simulink model "NN Controlled IM Drive"  (R2020b)
settings: Solver=ode4  StartTime=0.0  StopTime=5  RelTol=1e-3
InitFcn:
  | %clear;
  | %clc;
  | 
  | %Motor Parameters
  | r1 = 1.405;
  | l1  = 0.005839;
  | r2 = 1.395;
  | l2 = 0.005839;
  | Lm = 0.1722;
  | J = 0.0131;
  | 
  | %Motor Rated Values
  | Vrat = 400;
  | frat = 50;
  | 
  | x1 = 2*pi*frat*l1;
  | x2 = 2*pi*frat*l2;
  | Xm = 2*pi*frat*Lm;
  | Prat = 4*1000;
  | Nrat = 1430;
  | P = 4;
  | Ns = 120*frat/P;
  | nrat = Nrat*2*pi/60;
  | ns = Ns*2*pi/60;
  | srat = (Ns-Nrat)/Ns;
  | 
  | E1 = Vrat/sqrt(3); %phase voltage
  | IL = E1/( (r1 + (1i*x1) ) + ( ( (1i*x2) +(r2/srat) )*1i*Xm / ( (1i*Xm) + (1i*x2) + (r2/srat) ) ) );
  | E2 = E1 - (IL*(r1 + (1i*x1) ) );
  | Trat = (3/(ns))*srat*abs(E2)*abs(E2)*r2/((r2*r2) + (srat*srat*x2*x2));
  | %Trat = Prat/nrat;
  | 
  | %System Variables
  | Tsys = (1e-6);
  | Ts = (100e-6);
  | freq = 50;
  | ws = freq*2*pi;
  | 
  | m=1*freq/50;
  | %m = 1 * (freq/50);
  | Vbus = (400*sqrt(2)*2/sqrt(3)) / (1.15);
  | 
  | Vref = (Vbus*sqrt(3)/2) * m;
  | delay = Ts/Tsys;
  | 
  | % Motor Starting Parameters
  | inc_time = 0.1;
  | 
  | %Motor Loading time
  | load_time = 0;
  | 
  | %No. of Hybrid Zones
  | numzones = 3;
  | 
  | %Load ML model Weights
  | 
  | W1R_s1 = readmatrix('Regression Weights\W1_subnet1_tmp_odd_90.xlsx');
  | b1R_s1 = readmatrix('Regression Weights\b1_subnet1_tmp_odd_90.xlsx');
  | W1R_s2 = readmatrix('Regression Weights\W1_subnet2_tmp_odd_90.xlsx');
  | b1R_s2 = readmatrix('Regression Weights\b1_subnet2_tmp_odd_90.xlsx');
  | 
  | W2R = readmatrix('Regression Weights\W2_subnet_tmp_odd_90.xlsx');
  | b2R = readmatrix('Regression Weights\b2_subnet_tmp_odd_90.xlsx');
  | 
  | 
  | W1C_s1 = readmatrix('Classification Weights\W1_subnet1_tmp.xlsx');
  | b1C_s1 = readmatrix('Classification Weights\b1_subnet1_tmp.xlsx');
  | W1C_s2 = readmatrix('Classification Weights\W1_subnet2_tmp.xlsx');
  | b1C_s2 = readmatrix('Classification Weights\b1_subnet2_tmp.xlsx');
  | 
  | W2C = readmatrix('Classification Weights\W2_subnet_tmp.xlsx');
  | b2C = readmatrix('Classification Weights\b2_subnet_tmp.xlsx');
  | 
  | %For Vector Control
  | Ls = l1+Lm;
  | Lr = l2+Lm;
  | Tr = Ls/r2;
  | w_s = Ns*2*pi/60;
  | sigma = 1-(Lm*Lm/(Ls*Lr));
  | sigma_r = (Lr/Lm)-1;
  | G = 1;
  | 
  | %isd_star = 3.9346;
  | %isq_star = 7.5149;
  | w_star = nrat;
  | %phi_star = 0.7005;
  | 
  | T = (Prat/nrat);
  | isd_star = Vrat*sqrt(2/3)/sqrt((r1.^2)+((2*pi*frat*Ls).^2));
  | phi_star = Lm*isd_star;
  | cnst = (3/2)*(P/2)*(Lm*Lm/Lr)*isd_star;
  | isq_star = T/cnst;
  | 
  | %Load Controller NN Weights \tmp14_++
  | W1_c = readmatrix('Controller NN Weights\tmp14_++\W1.xlsx');
  | b1_c = readmatrix('Controller NN Weights\tmp14_++\b1.xlsx');
  | W2_c = readmatrix('Controller NN Weights\tmp14_++\W2.xlsx');
  | b2_c = readmatrix('Controller NN Weights\tmp14_++\b2.xlsx');
  | 
  | %Speed Control Loop
  | tau = 0.318e-3;
  | K_cont = (2/3)*(P/2)*(1/(1+sigma_r))*phi_star;
  | Ksp = J/(2*K_cont*tau);
  | Ksi = 1/(4*tau);
  | 
  | %ZOH Time
  | Tzoh = 1e-4;
undefined symbols (not defined in the file): DiscIntNeverNeededParam
libraries: powerlib x22, simulink x20, pid_lib x4, powerlib_meascontrol x3, simulink_extras x2
(part 1 of 3)
settings Model: Creator=hp  LastModifiedBy=hp
settings DataIOCC: ReturnWorkspaceOutputs=off

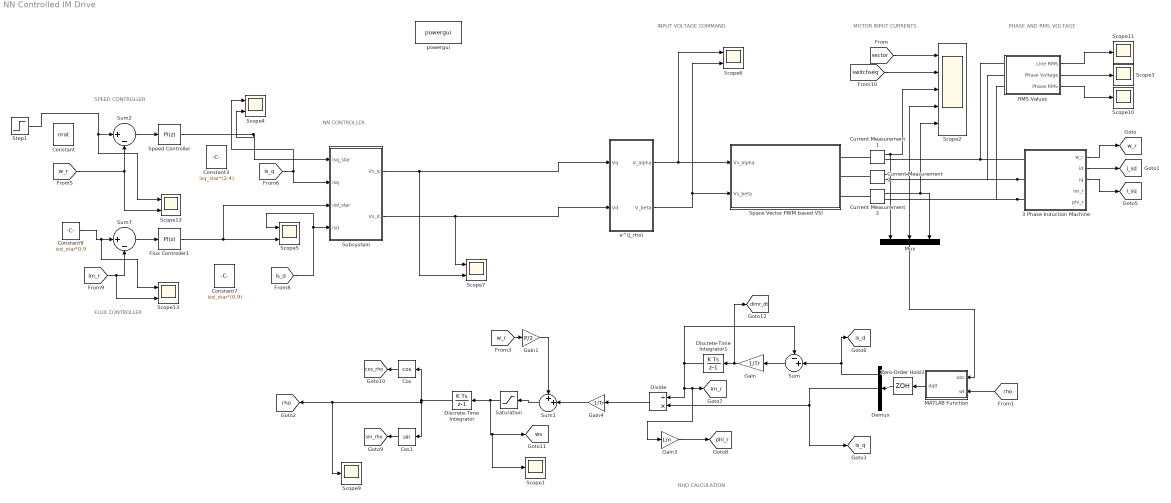
== system NN Controlled IM Drive ==
  note: PHASE AND RMS VOLTAGE
  note: MOTOR INPUT CURRENTS
  note: RHO CALCULATION
  note: INPUT VOLTAGE COMMAND
  note: NN CONTROLLER
  note: FLUX CONTROLLER
  note: SPEED CONTROLLER
  3 Phase Induction Machine : Subsystem
  Constant : Constant  Value=nrat
  Constant3 : Constant  Value=isq_star*(2.4)
  Constant7 : Constant  Value=isd_star*(0.9)
  Constant9 : Constant  Value=isd_star*0.9
  Cos : Trigonometry  Operator=cos
  Cos1 : Trigonometry
  Current Measurement1 : powerlib/Measurements/Current Measurement  PhasorSimulation=off  OutputType=Complex  PSBequivalent=0
  Current Measurement2 : powerlib/Measurements/Current Measurement  PhasorSimulation=off  OutputType=Complex  PSBequivalent=0
  Current Measurement3 : powerlib/Measurements/Current Measurement  PhasorSimulation=off  OutputType=Complex  PSBequivalent=0
  Demux : Demux  Outputs=3
  Discrete-Time Integrator : DiscreteIntegrator  SampleTime=-1  ICPrevOutput=DiscIntNeverNeededParam  ICPrevScaledInput=DiscIntNeverNeededParam
  Discrete-Time Integrator1 : DiscreteIntegrator  InitialCondition=1e-2  SampleTime=-1  ICPrevOutput=DiscIntNeverNeededParam  ICPrevScaledInput=DiscIntNeverNeededParam
  Divide : Product  Inputs=/*
  Flux Controller1 : pid_lib/PID Controller  Controller=PI  Form=Ideal  TimeDomain=Discrete-time  UseExternalTs=off  SampleTime=-1  IntegratorMethod=Forward Euler  FilterMethod=Forward Euler  ControllerParametersSource=internal  P=16*0.5*1.5/0.5  I=0.5*10/10  D=0  UseFilter=on  N=100  TunerSelectOption=Transfer Function Based (PID Tuner App)  InitialConditionSource=internal  InitialConditionForIntegrator=0  InitialConditionForFilter=0  DifferentiatorICPrevScaledInput=0  ExternalReset=none  TrackingMode=off  Kt=1  LimitOutput=on  SatLimitsSource=internal  UpperSaturationLimit=7  LowerSaturationLimit=-7  LinearizeAsGain=on  AntiWindupMode=none  Kb=1  POutMin=[]  POutMax=[]  IOutMin=[]  IOutMax=[]  DOutMin=[]  DOutMax=[]  NOutMin=[]  NOutMax=[]  SumOutMin=[]  SumOutMax=[]  SaturationOutMin=[]  SaturationOutMax=[]  PParamMin=[]  PParamMax=[]  IParamMin=[]  IParamMax=[]  DParamMin=[]  DParamMax=[]  NParamMin=[]  NParamMax=[]  KbParamMin=[]  KbParamMax=[]  KtParamMin=[]  KtParamMax=[]  KbOutMin=[]  KbOutMax=[]  KtOutMin=[]  KtOutMax=[]  IntegratorOutMin=[]  IntegratorOutMax=[]  FilterOutMin=[]  FilterOutMax=[]  SumI1OutMin=[]  SumI1OutMax=[]  SumI2OutMin=[]  SumI2OutMax=[]  SumI3OutMin=[]  SumI3OutMax=[]  SumI4OutMin=[]  SumI4OutMax=[]  SumDOutMin=[]  SumDOutMax=[]  DifferentiatorOutMin=[]  DifferentiatorOutMax=[]  FilterDiffOutCoefMin=[]  FilterDiffOutCoefMax=[]  ReciprocalOutMin=[]  ReciprocalOutMax=[]  SumDenOutMin=[]  SumDenOutMax=[]  SumNumOutMin=[]  SumNumOutMax=[]  DivideOutMin=[]  DivideOutMax=[]  UdiffTsProdOutMin=[]  UdiffTsProdOutMax=[]  NTsProdOutMin=[]  NTsProdOutMax=[]  UintegralTsProdOutMin=[]  UintegralTsProdOutMax=[]  UngainTsProdOutMin=[]  UngainTsProdOutMax=[]  IntegratorContinuousStateAttributes=''  IntegratorStateMustResolveToSignalObject=off  IntegratorRTWStateStorageClass=Auto  FilterContinuousStateAttributes=''  FilterStateMustResolveToSignalObject=off  FilterRTWStateStorageClass=Auto  ParallelPVariant=Passthrough  IdealPVariant=InternalParameters  IVariant=InternalParameters  DVariant=Disabled  IntegratorVariant=Discrete  SatVariant=Enabled  AWVariant=Passthrough  PCopyVariant=Disabled  TRVariant=Disabled  FdbkBlocksVariant=Forward  IdealPFdbkVariant=Disabled  SatFdbkVariant=Disabled  DerivativeFilterVariant=Disabled  NVariant=Disabled  NCopyVariant=Disabled_SignalSpec  FilterICVariant=Disabled  IntegratorICVariant=InternalICs  ExternalResetVariant=Disabled  TRSumVariant=Passthrough  SumFdbkVariant=Disabled  SumVariant=Sum_PI  TsampFilterVariant=InternalTs  TsampNgainVariant=Passthrough  TsampIntegralVariant=Passthrough  ExternalSaturationOutDataTypeStr=Inherit: Same as second input
  Gain : Gain  Gain=1/Tr
  Gain1 : Gain  Gain=P/2
  Gain3 : Gain  Gain=Lm
  Gain4 : Gain  Gain=1/Tr
  MATLAB Function : MATLAB Function  TreatAsAtomicUnit=on
  Mux : Mux  Inputs=3
  RMS Values : Subsystem
  Saturation : Saturate  UpperLimit=2*ws  LowerLimit=-2*ws
  Scope{1,3,9..11} (5 alike) : Scope
  Scope{4..7,12..13} (6 alike) : Scope  NumInputPorts=2
  Scope2 : Scope  NumInputPorts=5
  "Space Vector PWM based VSI " : Subsystem
  Speed Controller : pid_lib/PID Controller  Controller=PI  Form=Ideal  TimeDomain=Discrete-time  UseExternalTs=off  SampleTime=-1  IntegratorMethod=Forward Euler  FilterMethod=Forward Euler  ControllerParametersSource=internal  P=0.11*2/2  I=10*5/5  D=0  UseFilter=on  N=100  TunerSelectOption=Transfer Function Based (PID Tuner App)  InitialConditionSource=internal  InitialConditionForIntegrator=0  InitialConditionForFilter=0  DifferentiatorICPrevScaledInput=0  ExternalReset=none  TrackingMode=off  Kt=1  LimitOutput=on  SatLimitsSource=internal  UpperSaturationLimit=30  LowerSaturationLimit=-14  LinearizeAsGain=on  AntiWindupMode=none  Kb=1  POutMin=[]  POutMax=[]  IOutMin=[]  IOutMax=[]  DOutMin=[]  DOutMax=[]  NOutMin=[]  NOutMax=[]  SumOutMin=[]  SumOutMax=[]  SaturationOutMin=[]  SaturationOutMax=[]  PParamMin=[]  PParamMax=[]  IParamMin=[]  IParamMax=[]  DParamMin=[]  DParamMax=[]  NParamMin=[]  NParamMax=[]  KbParamMin=[]  KbParamMax=[]  KtParamMin=[]  KtParamMax=[]  KbOutMin=[]  KbOutMax=[]  KtOutMin=[]  KtOutMax=[]  IntegratorOutMin=[]  IntegratorOutMax=[]  FilterOutMin=[]  FilterOutMax=[]  SumI1OutMin=[]  SumI1OutMax=[]  SumI2OutMin=[]  SumI2OutMax=[]  SumI3OutMin=[]  SumI3OutMax=[]  SumI4OutMin=[]  SumI4OutMax=[]  SumDOutMin=[]  SumDOutMax=[]  DifferentiatorOutMin=[]  DifferentiatorOutMax=[]  FilterDiffOutCoefMin=[]  FilterDiffOutCoefMax=[]  ReciprocalOutMin=[]  ReciprocalOutMax=[]  SumDenOutMin=[]  SumDenOutMax=[]  SumNumOutMin=[]  SumNumOutMax=[]  DivideOutMin=[]  DivideOutMax=[]  UdiffTsProdOutMin=[]  UdiffTsProdOutMax=[]  NTsProdOutMin=[]  NTsProdOutMax=[]  UintegralTsProdOutMin=[]  UintegralTsProdOutMax=[]  UngainTsProdOutMin=[]  UngainTsProdOutMax=[]  IntegratorContinuousStateAttributes=''  IntegratorStateMustResolveToSignalObject=off  IntegratorRTWStateStorageClass=Auto  FilterContinuousStateAttributes=''  FilterStateMustResolveToSignalObject=off  FilterRTWStateStorageClass=Auto  ParallelPVariant=Passthrough  IdealPVariant=InternalParameters  IVariant=InternalParameters  DVariant=Disabled  IntegratorVariant=Discrete  SatVariant=Enabled  AWVariant=Passthrough  PCopyVariant=Disabled  TRVariant=Disabled  FdbkBlocksVariant=Forward  IdealPFdbkVariant=Disabled  SatFdbkVariant=Disabled  DerivativeFilterVariant=Disabled  NVariant=Disabled  NCopyVariant=Disabled_SignalSpec  FilterICVariant=Disabled  IntegratorICVariant=InternalICs  ExternalResetVariant=Disabled  TRSumVariant=Passthrough  SumFdbkVariant=Disabled  SumVariant=Sum_PI  TsampFilterVariant=InternalTs  TsampNgainVariant=Passthrough  TsampIntegralVariant=Passthrough  ExternalSaturationOutDataTypeStr=Inherit: Same as second input
  Step1 : Step  Time=0.5  After=nrat  SampleTime=0
  Subsystem : Subsystem
  Sum : Sum  Inputs=-+|
  Sum1 : Sum  Inputs=++|
  Sum2 : Sum  Inputs=|+-
  Sum7 : Sum  Inputs=|+-
  Zero-Order Hold3 : ZeroOrderHold  SampleTime=Tzoh
  e^(j_rho) : Subsystem
  powergui : powerlib/powergui  Priority=1  SimulationMode=Discrete  SampleTime=1e-6  frequency=60  Iterations=50  frequencyindice=50  Pbase=100e6  ErrMax=1e-4  UnitsV=kV  UnitsW=MW  buscounter=0  FunctionMessages=off  echomessages=off  EnableUseOfTLC=off  CurrentSourceSwitches=off  DisableSnubberDevices=off  DisableRonSwitches=off  DisableVfSwitches=off  DisplayEquations=off  AutomaticDiscreteSolvers=off  SolverType=Tustin/Backward Euler (TBE)  Interpol=off  ExternalGateDelay=off  methode=off  Ts=100  x0status=blocks  SPID=on  SwTol=0  HookPort=off  NonlinearTolerance=1e-4  nMaxIteration=100  ContinueOnMaxIteration=off  RestoreLinks=warning  ResistiveCurrentMeasurement=off  Frange=[0:2:500]  Ylog=off  Xlog=on  ShowGrid=off  save=off  variable=ZData  structure=ScopeData4  ZoomFFT=off  StartTime=1.4  cycles=1  DisplayStyle=1  fundamental=50  FreqAxis=off  MaxFrequency=1000  frequencyindicesteady=1  RmsSteady=1  display=off
  tag scope: cos_rho=global, dimr_dt=global, i_sd=global, i_sq=global, im_r=global, is_d=global, is_q=global, phi_r=global, rho=global, sin_rho=global, w_r=global, ws=global
  wires:
  Current Measurement2/1 -> Mux/2, Scope2/4
  3 Phase Induction Machine/1(w_r) -> [w_r]
  e^(j_rho)/2(V_beta) -> Scope6/2, "Space Vector PWM based VSI "/2(Vs_beta)
  Discrete-Time Integrator1/1 -> Sum/1, Gain3/1, [im_r], Divide/1
  [rho] -> MATLAB Function/2(wt)
  Mux/1 -> MATLAB Function/1(abc)
  [w_r] -> Gain1/1
  Demux/1 -> [is_d], Sum/2
  [switchseq] -> Scope2/2
  Gain/1 -> [dimr_dt], Discrete-Time Integrator1/1
  e^(j_rho)/1(V_alpha) -> Scope6/1, "Space Vector PWM based VSI "/1(Vs_alpha)
  Sum/1 -> Gain/1
  Demux/2 -> [is_q], Divide/2
  Current Measurement1/1 -> Scope2/3, Mux/1
  Cos1/1 -> [sin_rho]
  Current Measurement3/1 -> Mux/3, Scope2/5
  Gain1/1 -> Sum1/1
  [im_r] -> Scope13/2, Sum7/2
  [w_r] -> Sum2/2, Scope12/2
  RMS Values/1(Line RMS) -> Scope11/1
  Sum2/1 -> Speed Controller/1
  3 Phase Induction Machine/2(id) -> [i_sd]
  Sum7/1 -> Flux Controller1/1
  Discrete-Time Integrator/1 -> Scope9/1, [rho], Cos1/1, Cos/1
  3 Phase Induction Machine/3(iq) -> [i_sq]
  RMS Values/3(Phase RMS) -> Scope10/1
  RMS Values/2(Phase Voltage) -> Scope3/1
  Cos/1 -> [cos_rho]
  [sector] -> Scope2/1
  Sum1/1 -> Saturation/1
  Saturation/1 -> Scope1/1, [ws], Discrete-Time Integrator/1
  Constant9/1 -> Scope13/1, Sum7/1
  Step1/1 -> Scope12/1, Sum2/1
  Gain3/1 -> [phi_r]
  Gain4/1 -> Sum1/2
  Divide/1 -> Gain4/1
  MATLAB Function/1(dq0) -> Zero-Order Hold3/1
  [is_q] -> Scope4/1, Subsystem/2(isq)
  [is_d] -> Scope5/1, Subsystem/4(isd)
  Subsystem/2(Vs_d) -> e^(j_rho)/2(Vd), Scope7/1
  Subsystem/1(Vs_q) -> e^(j_rho)/1(Vq), Scope7/2
  Speed Controller/1 -> Scope4/2, Subsystem/1(isq_star)
  Flux Controller1/1 -> Subsystem/3(isd_star), Scope5/2
  Zero-Order Hold3/1 -> Demux/1
  connections:
  3 Phase Induction Machine/LConn2 -- RMS Values/LConn2 -- Current Measurement2/RConn1
  RMS Values/LConn1 -- Current Measurement1/RConn1 -- 3 Phase Induction Machine/LConn1
  3 Phase Induction Machine/LConn3 -- RMS Values/LConn3 -- Current Measurement3/RConn1
  Current Measurement1/LConn1 -- "Space Vector PWM based VSI "/RConn1
  Current Measurement3/LConn1 -- "Space Vector PWM based VSI "/RConn3
  Current Measurement2/LConn1 -- "Space Vector PWM based VSI "/RConn2

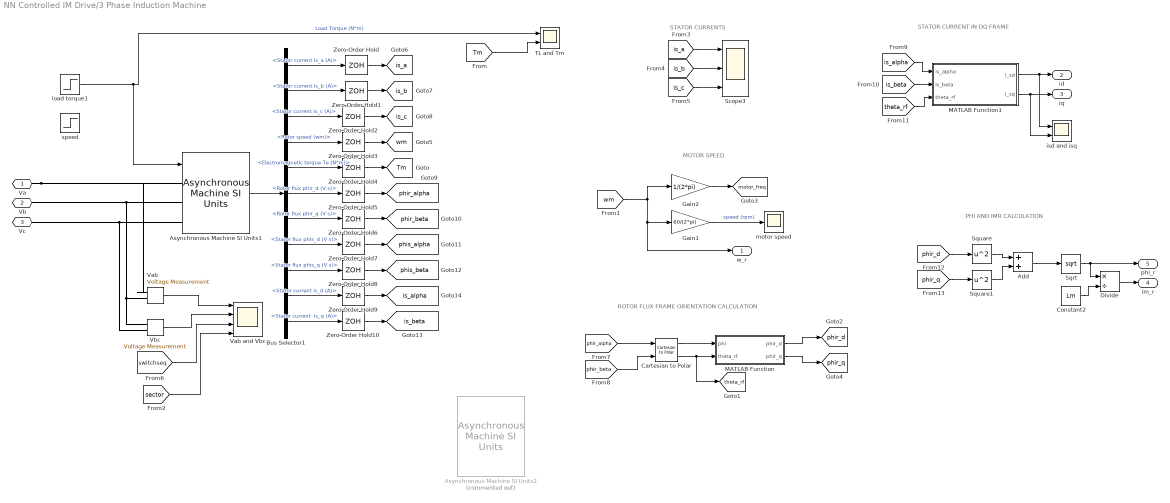
== system NN Controlled IM Drive/3 Phase Induction Machine ==
  note: MOTOR SPEED
  note: STATOR CURRENTS
  note: ROTOR FLUX FRAME ORIENTATION CALCULATION
  note: STATOR CURRENT IN DQ FRAME
  note: PHI AND IMR CALCULATION
  Add : Sum
  Asynchronous Machine SI Units1 : powerlib/Machines/Asynchronous Machine SI Units  RotorType=Squirrel-cage  PresetModel=No  MechanicalLoad=Torque Tm  ShowDetailedParameters=on  ReferenceFrame=Stationary  Units=SI  MeasurementBus=off  NominalParameters=[4000 400 50]  Stator=[1.405 0.005839]  Rotor=[1.395 0.005839]  Cage1=[0.4155 0.002066]  Cage2=[0.4168 0.0003495]  Lm=0.1722  Mechanical=[0.02 0.002985 2]  PolePairs=2  InitialConditions="[ 1,0   0,0,0   0,0,0 ]"  SimulateSaturation=off  Saturation=[14.03593122, 27.81365428, 53.79336849, 72.68890987, 97.98006896, 148.6815601, 215.7428561, 302.9841135, 428.7778367 ; 230, 322, 414, 460, 506, 552, 598, 644, 690]  LoadFlowParameters=1492000  TsPowergui=0  TsBlock=-1  IterativeModel=Trapezoidal non iterative  IterativeDiscreteModel=Trapezoidal non iterative  Pmec=0
  Asynchronous Machine SI Units2 : powerlib/Machines/Asynchronous Machine SI Units  Commented=on  RotorType=Squirrel-cage  PresetModel="15:  5.4 HP (4KW)   400 V  50Hz 1430 RPM"  MechanicalLoad=Torque Tm  ShowDetailedParameters=on  ReferenceFrame=Stationary  Units=SI  MeasurementBus=off  NominalParameters=[4000 400 50]  Stator=[1.405 0.005839]  Rotor=[1.395 0.005839]  Cage1=[0.4155 0.002066]  Cage2=[0.4168 0.0003495]  Lm=0.1722  Mechanical=[0.0131 0.002985 2]  PolePairs=2  InitialConditions="[ 1,0   0,0,0   0,0,0 ]"  SimulateSaturation=off  Saturation=[14.03593122, 27.81365428, 53.79336849, 72.68890987, 97.98006896, 148.6815601, 215.7428561, 302.9841135, 428.7778367 ; 230, 322, 414, 460, 506, 552, 598, 644, 690]  LoadFlowParameters=1492000  TsPowergui=0  TsBlock=-1  IterativeModel=Trapezoidal non iterative  IterativeDiscreteModel=Trapezoidal non iterative  Pmec=0
  Bus Selector1 : BusSelector  OutputSignals="Stator measurements.Stator current is_a (A),Stator measurements.Stator current is_b (A),Stator measurements.Stator current is_c (A),Mechanical.Rotor speed (wm),Mechanical.Electromagnetic torque Te (N*m),Rotor measurements.Rotor flux phir_d (V s),Rotor measurements.Rotor flux phir_q (V s),Stator measurements.Stator flux phis_d (V s),Stator measurements.Stator flux phis_q (V s),Stator measurements.Stator current is_d (A),Stator measurements.Stator current  is_q (A)"
  Cartesian to Polar : simulink_extras/Transformations/Cartesian to Polar
  Constant2 : Constant  Value=Lm
  Divide : Product  Inputs=*/
  Gain1 : Gain  Gain=60/(2*pi)
  Gain2 : Gain  Gain=1/(2*pi)
  MATLAB Function : MATLAB Function  TreatAsAtomicUnit=on
  MATLAB Function1 : MATLAB Function  TreatAsAtomicUnit=on
  Scope3 : Scope  NumInputPorts=3
  Sqrt : Sqrt  SaturateOnIntegerOverflow=on
  Square : Math  Operator=square  SaturateOnIntegerOverflow=on
  Square1 : Math  Operator=square  SaturateOnIntegerOverflow=on
  TL and Tm : Scope  NumInputPorts=2
  Vab : powerlib/Measurements/Voltage Measurement  PhasorSimulation=off  OutputType=Complex  PSBequivalent=0
  Vab and Vbc : Scope  NumInputPorts=4
  Vbc : powerlib/Measurements/Voltage Measurement  PhasorSimulation=off  OutputType=Complex  PSBequivalent=0
  Zero-Order Hold{,1..10} (11 alike) : ZeroOrderHold  SampleTime=Tzoh
  isd and isq : Scope  NumInputPorts=2
  load torque1 : Step  Time=3  After=T*0.5  SampleTime=Tsys
  motor speed : Scope
  speed : Step  Time=0  After=nrat  SampleTime=Tsys
  Va : PMIOPort  Side=Left
  Vb : PMIOPort  Port=2  Side=Left
  Vc : PMIOPort  Port=3  Side=Left
  w_r : Outport
  id : Outport  Port=2
  iq : Outport  Port=3
  im_r : Outport  Port=4
  phi_r : Outport  Port=5
  tag scope: Tm=global, is_a=global, is_alpha=global, is_b=global, is_beta=global, is_c=global, motor_freq=global, phir_alpha=global, phir_beta=global, phir_d=global, phir_q=global, phis_alpha=global, phis_beta=global, theta_rf=global, wm=global
  wires:
  load torque1/1 -> Asynchronous Machine SI Units1/1, TL and Tm/1  "Load Torque (N*m)"
  Asynchronous Machine SI Units1/1 -> Bus Selector1/1
  Gain1/1 -> motor speed/1  "speed (rpm)"
  Bus Selector1/5 -> Zero-Order Hold4/1  "<Electromagnetic torque Te (N*m)>"
  [Tm] -> TL and Tm/2
  Vbc/1 -> Vab and Vbc/2
  Vab/1 -> Vab and Vbc/1
  [sector] -> Vab and Vbc/4
  [switchseq] -> Vab and Vbc/3
  Gain2/1 -> [motor_freq]
  Square/1 -> Add/1
  Square1/1 -> Add/2
  Add/1 -> Sqrt/1
  Sqrt/1 -> phi_r/1, Divide/1
  Constant2/1 -> Divide/2
  Divide/1 -> im_r/1
  Cartesian to Polar/2 -> [theta_rf], MATLAB Function/2(theta_rf)
  Cartesian to Polar/1 -> MATLAB Function/1(phi)
  MATLAB Function/1(phir_d) -> [phir_d]
  MATLAB Function/2(phir_q) -> [phir_q]
  Bus Selector1/4 -> Zero-Order Hold3/1  "<Rotor speed (wm)>"
  Bus Selector1/1 -> Zero-Order Hold/1  "<Stator current is_a (A)>"
  Bus Selector1/2 -> Zero-Order Hold1/1  "<Stator current is_b (A)>"
  Bus Selector1/3 -> Zero-Order Hold2/1  "<Stator current is_c (A)>"
  [wm] -> Gain2/1, w_r/1, Gain1/1
  [is_a] -> Scope3/1
  [is_b] -> Scope3/2
  [is_c] -> Scope3/3
  Bus Selector1/6 -> Zero-Order Hold5/1  "<Rotor flux phir_d (V s)>"
  Bus Selector1/7 -> Zero-Order Hold6/1  "<Rotor flux phir_q (V s)>"
  Bus Selector1/8 -> Zero-Order Hold7/1  "<Stator flux phis_d (V s)>"
  Bus Selector1/9 -> Zero-Order Hold8/1  "<Stator flux phis_q (V s)>"
  Bus Selector1/10 -> Zero-Order Hold9/1  "<Stator current is_d (A)>"
  Bus Selector1/11 -> Zero-Order Hold10/1  "<Stator current  is_q (A)>"
  [phir_alpha] -> Cartesian to Polar/1
  [phir_beta] -> Cartesian to Polar/2
  [is_alpha] -> MATLAB Function1/1(is_alpha)
  [is_beta] -> MATLAB Function1/2(is_beta)
  [theta_rf] -> MATLAB Function1/3(theta_rf)
  MATLAB Function1/1(i_sd) -> isd and isq/1, id/1
  MATLAB Function1/2(i_sq) -> isd and isq/2, iq/1
  [phir_d] -> Square/1
  [phir_q] -> Square1/1
  Zero-Order Hold/1 -> [is_a]
  Zero-Order Hold3/1 -> [wm]
  Zero-Order Hold2/1 -> [is_c]
  Zero-Order Hold1/1 -> [is_b]
  Zero-Order Hold10/1 -> [is_beta]
  Zero-Order Hold5/1 -> [phir_alpha]
  Zero-Order Hold7/1 -> [phis_alpha]
  Zero-Order Hold4/1 -> [Tm]
  Zero-Order Hold6/1 -> [phir_beta]
  Zero-Order Hold9/1 -> [is_alpha]
  Zero-Order Hold8/1 -> [phis_beta]
  connections:
  Vab/LConn2 -- Vb/RConn1 -- Asynchronous Machine SI Units1/LConn2 -- Vbc/LConn1
  Va/RConn1 -- Vab/LConn1 -- Asynchronous Machine SI Units1/LConn1
  Vc/RConn1 -- Vbc/LConn2 -- Asynchronous Machine SI Units1/LConn3

== system NN Controlled IM Drive/RMS Values ==
  Add : Sum  Inputs=+-
  Gain : Gain  Gain=1/3
  RMS1 : powerlib_meascontrol/Measurements/RMS  TrueRMS=off  Freq=50  RMSInit=0  Ts=Tsys
  RMS2 : powerlib_meascontrol/Measurements/RMS  TrueRMS=off  Freq=freq  RMSInit=0  Ts=Tsys
  Voltage Measurement : powerlib/Measurements/Voltage Measurement  PhasorSimulation=off  OutputType=Complex  PSBequivalent=0
  Voltage Measurement1 : powerlib/Measurements/Voltage Measurement  PhasorSimulation=off  OutputType=Complex  PSBequivalent=0
  Va : PMIOPort  Side=Left
  Vb : PMIOPort  Port=2  Side=Left
  Vc : PMIOPort  Port=3  Side=Left
  Line RMS : Outport
  Phase Voltage : Outport  Port=2
  Phase RMS : Outport  Port=3
  wires:
  Gain/1 -> Phase Voltage/1, RMS1/1
  Voltage Measurement/1 -> RMS2/1, Add/1
  Voltage Measurement1/1 -> Add/2
  RMS1/1 -> Phase RMS/1
  Add/1 -> Gain/1
  RMS2/1 -> Line RMS/1
  connections:
  Voltage Measurement1/LConn2 -- Va/RConn1 -- Voltage Measurement/LConn1
  Voltage Measurement1/LConn1 -- Vc/RConn1
  Voltage Measurement/LConn2 -- Vb/RConn1

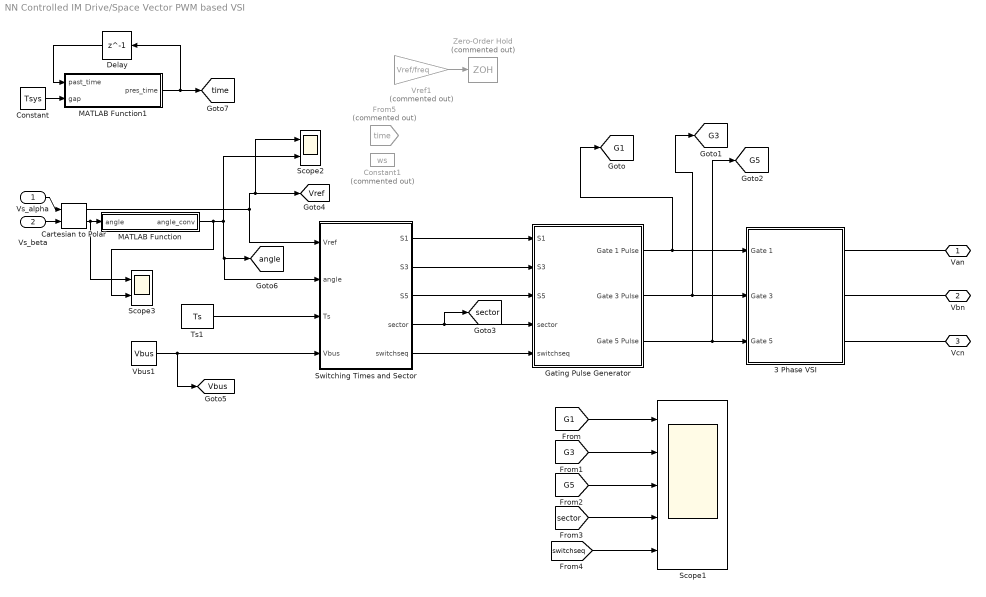
== system NN Controlled IM Drive/Space Vector PWM based VSI  ==
  Vs_alpha : Inport
  Vs_beta : Inport  Port=2
  3 Phase VSI : Subsystem
  Cartesian to Polar : simulink_extras/Transformations/Cartesian to Polar
  Constant : Constant  Value=Tsys
  Constant1 : Constant  Commented=on  Value=ws
  Delay : Delay  DelayLength=1
  From5 : From  Commented=on  GotoTag=time  TagVisibility=global
  Gating Pulse Generator : Subsystem
  MATLAB Function : MATLAB Function  TreatAsAtomicUnit=on
  MATLAB Function1 : MATLAB Function  TreatAsAtomicUnit=on
  Scope1 : Scope  NumInputPorts=5
  Scope2 : Scope  NumInputPorts=2
  Scope3 : Scope  NumInputPorts=2
  Switching Times and Sector : Subsystem
  Ts1 : Constant  Value=Ts  SampleTime=Tsys
  Vbus1 : Constant  Value=Vbus  SampleTime=Tsys
  Vref1 : Gain  Commented=on  Gain=Vref/freq
  Zero-Order Hold : ZeroOrderHold  Commented=on  SampleTime=Ts
  Van : PMIOPort  Side=Right
  Vbn : PMIOPort  Port=2  Side=Right
  Vcn : PMIOPort  Port=3  Side=Right
  tag scope: G1=global, G3=global, G5=global, Vbus=global, Vref=global, angle=global, sector=global, time=global
  wires:
  Switching Times and Sector/1(S1) -> Gating Pulse Generator/1(S1)
  Switching Times and Sector/2(S3) -> Gating Pulse Generator/2(S3)
  Switching Times and Sector/3(S5) -> Gating Pulse Generator/3(S5)
  Switching Times and Sector/4(sector) -> Gating Pulse Generator/4(sector), [sector]
  Switching Times and Sector/5(switchseq) -> Gating Pulse Generator/5(switchseq)
  Gating Pulse Generator/1(Gate 1 Pulse) -> [G1], 3 Phase VSI/1(Gate 1)
  Gating Pulse Generator/2(Gate 3 Pulse) -> [G3], 3 Phase VSI/2(Gate 3)
  Gating Pulse Generator/3(Gate 5 Pulse) -> [G5], 3 Phase VSI/3(Gate 5)
  [G1] -> Scope1/1
  [G3] -> Scope1/2
  [G5] -> Scope1/3
  [sector] -> Scope1/4
  [switchseq] -> Scope1/5
  Vref1/1 -> Zero-Order Hold/1
  Vbus1/1 -> [Vbus], Switching Times and Sector/4(Vbus)
  Ts1/1 -> Switching Times and Sector/3(Ts)
  Vs_beta/1 -> Cartesian to Polar/2
  Vs_alpha/1 -> Cartesian to Polar/1
  Cartesian to Polar/1 -> Switching Times and Sector/1(Vref), Scope2/1, [Vref]
  MATLAB Function1/1(pres_time) -> Delay/1, [time]
  Delay/1 -> MATLAB Function1/1(past_time)
  Constant/1 -> MATLAB Function1/2(gap)
  Cartesian to Polar/2 -> Scope3/1, MATLAB Function/1(angle)
  MATLAB Function/1(angle_conv) -> Scope3/2, Switching Times and Sector/2(angle), [angle], Scope2/2
  connections:
  Vbn/RConn1 -- 3 Phase VSI/RConn2
  Vcn/RConn1 -- 3 Phase VSI/RConn3
  3 Phase VSI/RConn1 -- Van/RConn1

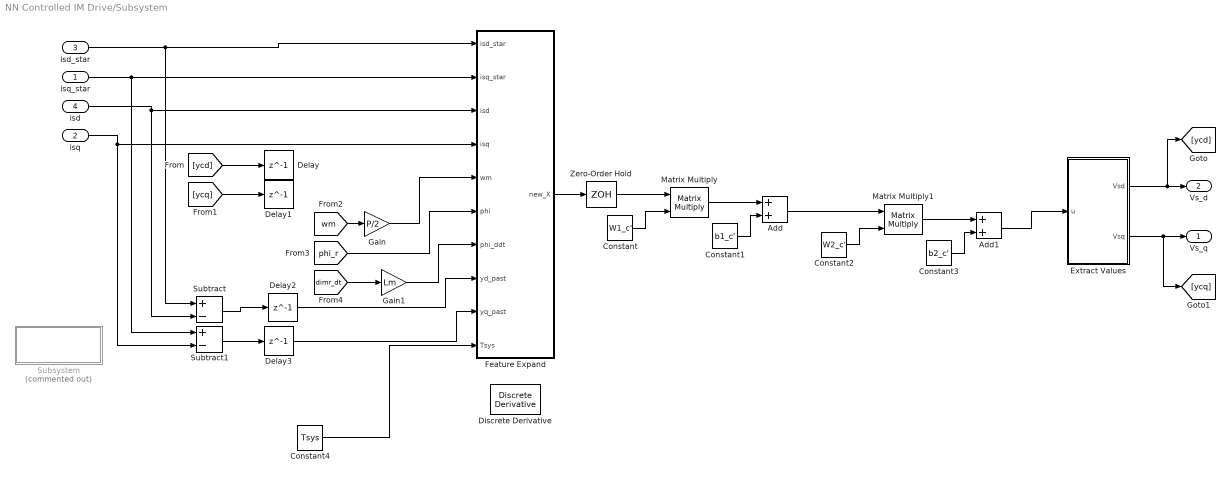
== system NN Controlled IM Drive/Subsystem ==
  isq_star : Inport
  isq : Inport  Port=2
  isd_star : Inport  Port=3
  isd : Inport  Port=4
  Add : Sum
  Add1 : Sum
  Constant : Constant  Value=W1_c'
  Constant1 : Constant  Value=b1_c'
  Constant2 : Constant  Value=W2_c'
  Constant3 : Constant  Value=b2_c'
  Constant4 : Constant  Value=Tsys
  Delay : Delay  DelayLength=1
  Delay1 : Delay  DelayLength=1
  Delay2 : Delay  DelayLength=1  SampleTime=50e-6
  Delay3 : Delay  DelayLength=1  SampleTime=50e-6
  Discrete Derivative : simulink/Discrete/Discrete Derivative  gainval=1.0  ICPrevScaledInput=0.0  OutMin=[]  OutMax=[]  OutDataType=fixdt(1, 16)  OutScaling=2^-10  DoSatur=off
  Extract Values : MATLAB Function  TreatAsAtomicUnit=on
  Feature Expand : MATLAB Function  TreatAsAtomicUnit=on
  Gain : Gain  Gain=P/2
  Gain1 : Gain  Gain=Lm
  Matrix Multiply : Product  Multiplication=Matrix(*)
  Matrix Multiply1 : Product  Multiplication=Matrix(*)
  Subsystem : Subsystem  Commented=on
  Subtract : Sum  Inputs=+-
  Subtract1 : Sum  Inputs=+-
  Zero-Order Hold : ZeroOrderHold  SampleTime=Ts
  Vs_q : Outport
  Vs_d : Outport  Port=2
  wires:
  Matrix Multiply/1 -> Add/1
  Constant1/1 -> Add/2
  Constant/1 -> Matrix Multiply/2
  isq_star/1 -> Subtract1/1, Feature Expand/2(isq_star)
  isd_star/1 -> Subtract/1, Feature Expand/1(isd_star)
  isd/1 -> Subtract/2, Feature Expand/3(isd)
  isq/1 -> Subtract1/2, Feature Expand/4(isq)
  [wm] -> Gain/1
  Gain/1 -> Feature Expand/5(wm)
  [phi_r] -> Feature Expand/6(phi)
  [dimr_dt] -> Gain1/1
  Extract Values/1(Vsd) -> Vs_d/1, [ycd]
  Extract Values/2(Vsq) -> [ycq], Vs_q/1
  Gain1/1 -> Feature Expand/7(phi_ddt)
  [ycd] -> Delay/1
  [ycq] -> Delay1/1
  Subtract/1 -> Delay2/1
  Subtract1/1 -> Delay3/1
  Constant2/1 -> Matrix Multiply1/2
  Matrix Multiply1/1 -> Add1/1
  Add/1 -> Matrix Multiply1/1
  Constant3/1 -> Add1/2
  Add1/1 -> Extract Values/1(u)
  Delay2/1 -> Feature Expand/8(yd_past)
  Delay3/1 -> Feature Expand/9(yq_past)
  Feature Expand/1(new_X) -> Zero-Order Hold/1
  Zero-Order Hold/1 -> Matrix Multiply/1
  Constant4/1 -> Feature Expand/10(Tsys)

== system NN Controlled IM Drive/e^(j_rho) ==
  Vq : Inport
  Vd : Inport  Port=2
  Add : Sum  Inputs=+-
  Add1 : Sum
  Product{,1..3} (4 alike) : Product
  V_alpha : Outport
  V_beta : Outport  Port=2
  wires:
  Vd/1 -> Product2/1, Product/1
  Vq/1 -> Product3/1, Product1/1
  Product/1 -> Add/1
  Product1/1 -> Add/2
  Add/1 -> V_alpha/1
  Product2/1 -> Add1/1
  Product3/1 -> Add1/2
  Add1/1 -> V_beta/1
  [cos_rho] -> Product/2, Product3/2
  [sin_rho] -> Product2/2, Product1/2

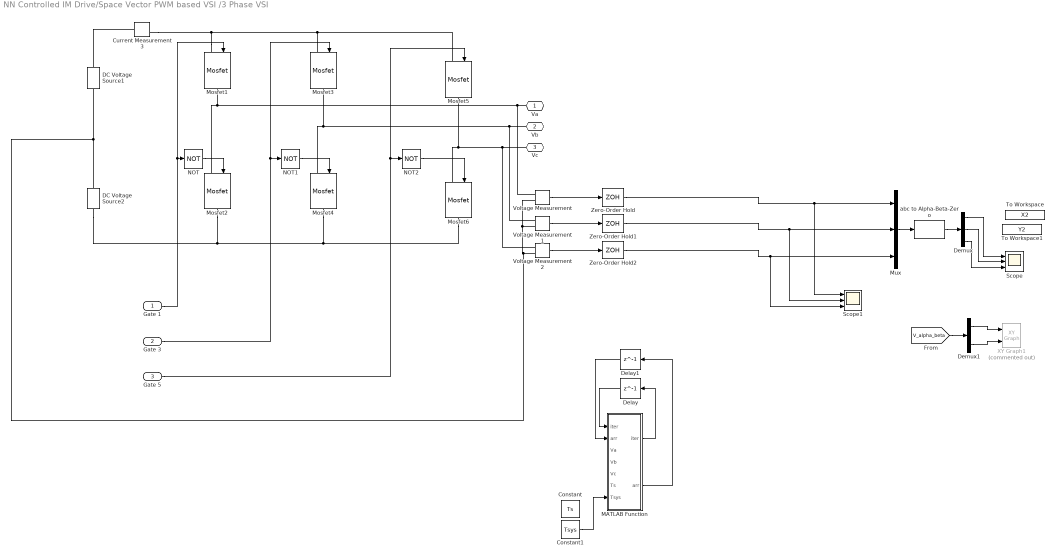
== system NN Controlled IM Drive/Space Vector PWM based VSI /3 Phase VSI ==
  Gate 1 : Inport
  Gate 3 : Inport  Port=2
  Gate 5 : Inport  Port=3
  Constant : Constant  Value=Ts  SampleTime=Tsys
  Constant1 : Constant  Value=Tsys  SampleTime=Tsys
  Current Measurement3 : powerlib/Measurements/Current Measurement  PhasorSimulation=off  OutputType=Complex  PSBequivalent=0
  DC Voltage Source1 : powerlib/Electrical Sources/DC Voltage Source  Amplitude=Vbus/2  Measurements=None
  DC Voltage Source2 : powerlib/Electrical Sources/DC Voltage Source  Amplitude=Vbus/2  Measurements=None
  Delay : Delay  DelayLength=1  SampleTime=Tsys
  Delay1 : Delay  DelayLength=1  SampleTime=Tsys
  Demux : Demux  Outputs=3
  Demux1 : Demux  Outputs=2
  MATLAB Function : MATLAB Function  TreatAsAtomicUnit=on
  Mosfet{1..6} (6 alike) : powerlib/Power Electronics/Mosfet  Ron=1e-6  Lon=0  Rd=1e-6  Vfd=0  IC=0  Rs=1e5  Cs=inf  Measurements=off
  Mux : Mux  Inputs=3
  NOT : Logic  Operator=NOT  IconShape=distinctive  AllPortsSameDT=off  OutDataTypeStr=boolean
  NOT1 : Logic  Operator=NOT  IconShape=distinctive  AllPortsSameDT=off  OutDataTypeStr=boolean
  NOT2 : Logic  Operator=NOT  IconShape=distinctive  AllPortsSameDT=off  OutDataTypeStr=boolean
  Scope : Scope  NumInputPorts=3
  Scope1 : Scope  NumInputPorts=3
  To Workspace : ToWorkspace  VariableName=X2  SampleTime=-1
  To Workspace1 : ToWorkspace  VariableName=Y2  SampleTime=-1
  Voltage Measurement : powerlib/Measurements/Voltage Measurement  PhasorSimulation=off  OutputType=Complex  PSBequivalent=0
  Voltage Measurement1 : powerlib/Measurements/Voltage Measurement  PhasorSimulation=off  OutputType=Complex  PSBequivalent=0
  Voltage Measurement2 : powerlib/Measurements/Voltage Measurement  PhasorSimulation=off  OutputType=Complex  PSBequivalent=0
  XY Graph1 : simulink/Sinks/XY Graph  Commented=on  xmin=-Vref  xmax=Vref  ymin=-Vref  ymax=Vref  st=Ts
  Zero-Order Hold : ZeroOrderHold  SampleTime=Ts
  Zero-Order Hold1 : ZeroOrderHold  SampleTime=Ts
  Zero-Order Hold2 : ZeroOrderHold  SampleTime=Ts
  abc to Alpha-Beta-Zero : powerlib_meascontrol/Transformations/abc to Alpha-Beta-Zero
  Va : PMIOPort  Side=Right
  Vb : PMIOPort  Port=2  Side=Right
  Vc : PMIOPort  Port=3  Side=Right
  wires:
  Gate 3/1 -> NOT1/1, Mosfet3/1
  NOT1/1 -> Mosfet4/1
  Gate 1/1 -> NOT/1, Mosfet1/1
  Gate 5/1 -> NOT2/1, Mosfet5/1
  NOT/1 -> Mosfet2/1
  NOT2/1 -> Mosfet6/1
  Mux/1 -> abc to Alpha-Beta-Zero/1
  abc to Alpha-Beta-Zero/1 -> Demux/1
  Demux/1 -> Scope/1
  Demux/2 -> Scope/2
  Demux/3 -> Scope/3
  [V_alpha_beta] -> Demux1/1
  Demux1/1 -> XY Graph1/1
  Demux1/2 -> XY Graph1/2
  Constant1/1 -> MATLAB Function/7(Tsys)
  MATLAB Function/1(iter) -> Delay/1
  Delay/1 -> MATLAB Function/1("iter ")
  Delay1/1 -> MATLAB Function/2("arr ")
  MATLAB Function/2(arr) -> Delay1/1
  Voltage Measurement/1 -> Zero-Order Hold/1
  Voltage Measurement1/1 -> Zero-Order Hold1/1
  Voltage Measurement2/1 -> Zero-Order Hold2/1
  Zero-Order Hold/1 -> Scope1/1, Mux/1
  Zero-Order Hold1/1 -> Scope1/2, Mux/2
  Zero-Order Hold2/1 -> Scope1/3, Mux/3
  connections:
  Mosfet6/LConn1 -- Voltage Measurement2/LConn1 -- Vc/RConn1 -- Mosfet5/RConn1
  Mosfet4/LConn1 -- Voltage Measurement1/LConn1 -- Vb/RConn1 -- Mosfet3/RConn1
  Current Measurement3/LConn1 -- DC Voltage Source1/RConn1
  Mosfet1/LConn1 -- Current Measurement3/RConn1 -- Mosfet5/LConn1 -- Mosfet3/LConn1
  Mosfet2/LConn1 -- Voltage Measurement/LConn1 -- Va/RConn1 -- Mosfet1/RConn1
  Mosfet4/RConn1 -- DC Voltage Source2/LConn1 -- Mosfet2/RConn1 -- Mosfet6/RConn1
  DC Voltage Source2/RConn1 -- DC Voltage Source1/LConn1 -- Voltage Measurement1/LConn2 -- Voltage Measurement/LConn2 -- Voltage Measurement2/LConn2

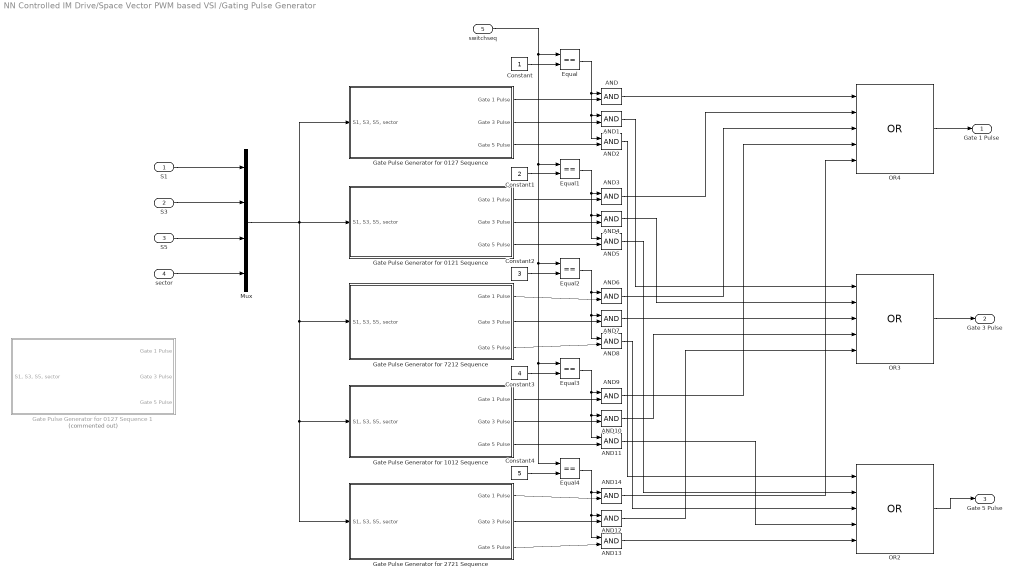
== system NN Controlled IM Drive/Space Vector PWM based VSI /Gating Pulse Generator ==
  S1 : Inport
  S3 : Inport  Port=2
  S5 : Inport  Port=3
  sector : Inport  Port=4
  switchseq : Inport  Port=5
  AND{,1..14} (15 alike) : Logic  IconShape=distinctive  AllPortsSameDT=off  OutDataTypeStr=boolean
  Constant : Constant
  Constant1 : Constant  Value=2
  Constant2 : Constant  Value=3
  Constant3 : Constant  Value=4
  Constant4 : Constant  Value=5
  Equal{,1..4} (5 alike) : RelationalOperator  Operator===  OutDataTypeStr=boolean  RndMeth=Simplest
  Gate Pulse Generator for 0121 Sequence : Subsystem
  Gate Pulse Generator for 0127 Sequence : Subsystem
  Gate Pulse Generator for 0127 Sequence 1 : Subsystem  Commented=on
  Gate Pulse Generator for 1012 Sequence : Subsystem
  Gate Pulse Generator for 2721 Sequence : Subsystem
  Gate Pulse Generator for 7212 Sequence : Subsystem
  Mux : Mux
  OR2 : Logic  Operator=OR  Inputs=5  IconShape=distinctive  AllPortsSameDT=off  OutDataTypeStr=boolean
  OR3 : Logic  Operator=OR  Inputs=5  IconShape=distinctive  AllPortsSameDT=off  OutDataTypeStr=boolean
  OR4 : Logic  Operator=OR  Inputs=5  IconShape=distinctive  AllPortsSameDT=off  OutDataTypeStr=boolean
  Gate 1 Pulse : Outport
  Gate 3 Pulse : Outport  Port=2
  Gate 5 Pulse : Outport  Port=3
  wires:
  sector/1 -> Mux/4
  S5/1 -> Mux/3
  S3/1 -> Mux/2
  S1/1 -> Mux/1
  Mux/1 -> Gate Pulse Generator for 0121 Sequence/1("S1, S3, S5, sector"), Gate Pulse Generator for 0127 Sequence/1("S1, S3, S5, sector"), Gate Pulse Generator for 7212 Sequence/1("S1, S3, S5, sector"), Gate Pulse Generator for 2721 Sequence/1("S1, S3, S5, sector"), Gate Pulse Generator for 1012 Sequence/1("S1, S3, S5, sector")
  Constant/1 -> Equal/2
  Equal/1 -> AND2/1, AND1/1, AND/1
  Gate Pulse Generator for 0121 Sequence/3(Gate 5 Pulse) -> AND5/2
  Gate Pulse Generator for 0121 Sequence/2(Gate 3 Pulse) -> AND4/2
  Equal1/1 -> AND3/1, AND4/1, AND5/1
  Gate Pulse Generator for 0121 Sequence/1(Gate 1 Pulse) -> AND3/2
  Constant1/1 -> Equal1/2
  Constant2/1 -> Equal2/2
  Gate Pulse Generator for 7212 Sequence/1(Gate 1 Pulse) -> AND6/2
  Equal2/1 -> AND8/1, AND7/1, AND6/1
  Gate Pulse Generator for 7212 Sequence/2(Gate 3 Pulse) -> AND7/2
  Gate Pulse Generator for 7212 Sequence/3(Gate 5 Pulse) -> AND8/2
  OR2/1 -> Gate 5 Pulse/1
  OR3/1 -> Gate 3 Pulse/1
  OR4/1 -> Gate 1 Pulse/1
  Gate Pulse Generator for 1012 Sequence/3(Gate 5 Pulse) -> AND11/2
  Gate Pulse Generator for 1012 Sequence/2(Gate 3 Pulse) -> AND10/2
  Equal3/1 -> AND10/1, AND11/1, AND9/1
  Gate Pulse Generator for 1012 Sequence/1(Gate 1 Pulse) -> AND9/2
  Constant3/1 -> Equal3/2
  switchseq/1 -> Equal/1, Equal4/1, Equal3/1, Equal2/1, Equal1/1
  Constant4/1 -> Equal4/2
  Gate Pulse Generator for 2721 Sequence/1(Gate 1 Pulse) -> AND14/2
  Equal4/1 -> AND14/1, AND13/1, AND12/1
  Gate Pulse Generator for 2721 Sequence/2(Gate 3 Pulse) -> AND12/2
  Gate Pulse Generator for 2721 Sequence/3(Gate 5 Pulse) -> AND13/2
  AND/1 -> OR4/1
  AND7/1 -> OR3/3
  AND13/1 -> OR2/5
  AND14/1 -> OR4/5
  AND3/1 -> OR4/2
  AND6/1 -> OR4/3
  AND9/1 -> OR4/4
  AND1/1 -> OR3/1
  AND4/1 -> OR3/2
  AND10/1 -> OR3/4
  AND12/1 -> OR3/5
  AND2/1 -> OR2/1
  AND5/1 -> OR2/2
  AND8/1 -> OR2/3
  AND11/1 -> OR2/4
  Gate Pulse Generator for 0127 Sequence/3(Gate 5 Pulse) -> AND2/2
  Gate Pulse Generator for 0127 Sequence/2(Gate 3 Pulse) -> AND1/2
  Gate Pulse Generator for 0127 Sequence/1(Gate 1 Pulse) -> AND/2

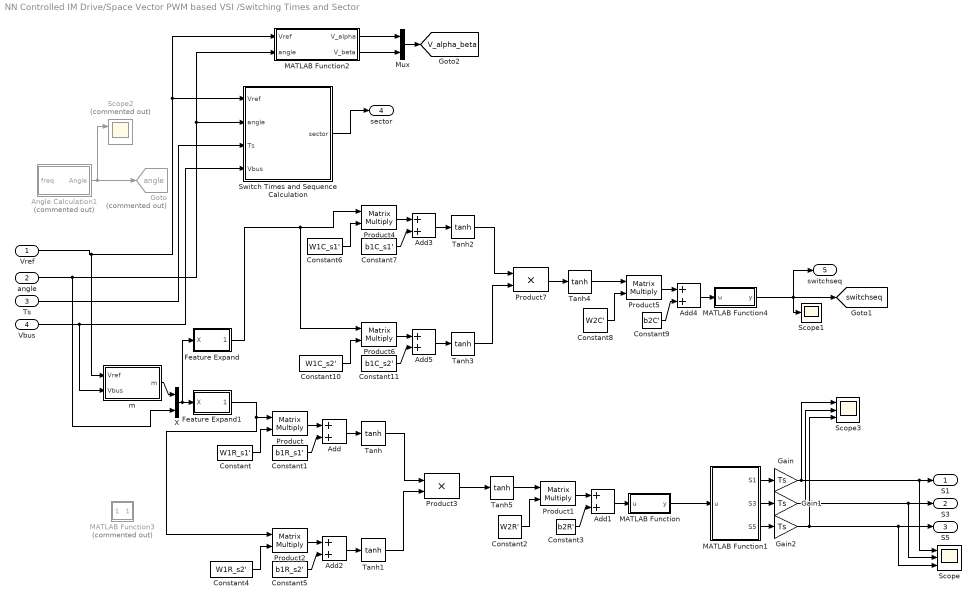
== system NN Controlled IM Drive/Space Vector PWM based VSI /Switching Times and Sector ==
  Vref : Inport
  angle : Inport  Port=2
  Ts : Inport  Port=3
  Vbus : Inport  Port=4
  Add{,1..5} (6 alike) : Sum
  Angle Calculation1 : Subsystem  Commented=on
  Constant : Constant  Value=W1R_s1'
  Constant1 : Constant  Value=b1R_s1'
  Constant10 : Constant  Value=W1C_s2'
  Constant11 : Constant  Value=b1C_s2'
  Constant2 : Constant  Value=W2R'
  Constant3 : Constant  Value=b2R'
  Constant4 : Constant  Value=W1R_s2'
  Constant5 : Constant  Value=b1R_s2'
  Constant6 : Constant  Value=W1C_s1'
  Constant7 : Constant  Value=b1C_s1'
  Constant8 : Constant  Value=W2C'
  Constant9 : Constant  Value=b2C'
  Feature Expand : MATLAB Function  TreatAsAtomicUnit=on
  Feature Expand1 : MATLAB Function  TreatAsAtomicUnit=on
  Gain : Gain  Gain=Ts
  Gain1 : Gain  Gain=Ts
  Gain2 : Gain  Gain=Ts
  Goto : Goto  Commented=on  GotoTag=angle  TagVisibility=global
  MATLAB Function : MATLAB Function  TreatAsAtomicUnit=on
  MATLAB Function1 : MATLAB Function  TreatAsAtomicUnit=on
  MATLAB Function2 : MATLAB Function  TreatAsAtomicUnit=on
  MATLAB Function3 : MATLAB Function  Commented=on  TreatAsAtomicUnit=on
  MATLAB Function4 : MATLAB Function  TreatAsAtomicUnit=on
  Mux : Mux  Inputs=2
  Product{,1..2,4..6} (6 alike) : Product  Multiplication=Matrix(*)
  Product3 : Product
  Product7 : Product
  Scope : Scope  NumInputPorts=3
  Scope1 : Scope
  Scope2 : Scope  Commented=on  NumInputPorts=2
  Scope3 : Scope  NumInputPorts=3
  Switch Times and Sequence Calculation : MATLAB Function  TreatAsAtomicUnit=on
  Tanh{,1..5} (6 alike) : Trigonometry  Operator=tanh
  X : Concatenate
  m : MATLAB Function  TreatAsAtomicUnit=on
  S1 : Outport
  S3 : Outport  Port=2
  S5 : Outport  Port=3
  sector : Outport  Port=4
  switchseq : Outport  Port=5
  tag scope: V_alpha_beta=global, switchseq=global
  wires:
  Vref/1 -> m/1(Vref), MATLAB Function2/1(Vref), Switch Times and Sequence Calculation/1(Vref)
  Ts/1 -> Switch Times and Sequence Calculation/3(Ts)
  angle/1 -> X/2, MATLAB Function2/2(angle), Switch Times and Sequence Calculation/2(angle)
  Switch Times and Sequence Calculation/1(sector) -> sector/1
  Constant/1 -> Product/2
  Product/1 -> Add/1
  Constant1/1 -> Add/2
  Constant3/1 -> Add1/2
  Product1/1 -> Add1/1
  Constant2/1 -> Product1/2
  Add/1 -> Tanh/1
  Add1/1 -> MATLAB Function/1(u)
  MATLAB Function/1(y) -> MATLAB Function1/1(u)
  X/1 -> Feature Expand/1(X), Feature Expand1/1(X)
  Angle Calculation1/1(Angle) -> Scope2/1, Goto/1
  MATLAB Function1/1(S1) -> Gain/1
  MATLAB Function1/3(S5) -> Gain2/1
  MATLAB Function1/2(S3) -> Gain1/1
  m/1(m) -> X/1
  Vbus/1 -> m/2(Vbus), Switch Times and Sequence Calculation/4(Vbus)
  Add2/1 -> Tanh1/1
  Constant5/1 -> Add2/2
  Product2/1 -> Add2/1
  Constant4/1 -> Product2/2
  Tanh1/1 -> Product3/2
  Tanh/1 -> Product3/1
  MATLAB Function2/1(V_alpha) -> Mux/1
  MATLAB Function2/2(V_beta) -> Mux/2
  Mux/1 -> [V_alpha_beta]
  Tanh2/1 -> Product7/1
  Tanh3/1 -> Product7/2
  Constant10/1 -> Product6/2
  Product6/1 -> Add5/1
  Constant11/1 -> Add5/2
  Add5/1 -> Tanh3/1
  Feature Expand/1(new_X) -> Product4/1, Product6/1
  MATLAB Function4/1(y) -> switchseq/1, Scope1/1, [switchseq]
  Add4/1 -> MATLAB Function4/1(u)
  Add3/1 -> Tanh2/1
  Constant8/1 -> Product5/2
  Product5/1 -> Add4/1
  Constant9/1 -> Add4/2
  Constant7/1 -> Add3/2
  Product4/1 -> Add3/1
  Constant6/1 -> Product4/2
  Product7/1 -> Tanh4/1
  Tanh4/1 -> Product5/1
  Tanh5/1 -> Product1/1
  Product3/1 -> Tanh5/1
  Feature Expand1/1(new_X) -> Product/1, Product2/1
  Gain/1 -> Scope/1, S1/1, Scope3/1
  Gain1/1 -> Scope/2, S3/1, Scope3/2
  Gain2/1 -> Scope/3, S5/1, Scope3/3

== system NN Controlled IM Drive/Subsystem/Subsystem ==
  Current Controller1 : pid_lib/PID Controller  Controller=PI  Form=Ideal  TimeDomain=Discrete-time  UseExternalTs=off  SampleTime=-1  IntegratorMethod=Forward Euler  FilterMethod=Forward Euler  ControllerParametersSource=internal  P=10  I=5  D=0  UseFilter=on  N=100  TunerSelectOption=Transfer Function Based (PID Tuner App)  InitialConditionSource=internal  InitialConditionForIntegrator=0  InitialConditionForFilter=0  DifferentiatorICPrevScaledInput=0  ExternalReset=none  TrackingMode=off  Kt=1  LimitOutput=on  SatLimitsSource=internal  UpperSaturationLimit=500  LowerSaturationLimit=-500  LinearizeAsGain=on  AntiWindupMode=none  Kb=1  POutMin=[]  POutMax=[]  IOutMin=[]  IOutMax=[]  DOutMin=[]  DOutMax=[]  NOutMin=[]  NOutMax=[]  SumOutMin=[]  SumOutMax=[]  SaturationOutMin=[]  SaturationOutMax=[]  PParamMin=[]  PParamMax=[]  IParamMin=[]  IParamMax=[]  DParamMin=[]  DParamMax=[]  NParamMin=[]  NParamMax=[]  KbParamMin=[]  KbParamMax=[]  KtParamMin=[]  KtParamMax=[]  KbOutMin=[]  KbOutMax=[]  KtOutMin=[]  KtOutMax=[]  IntegratorOutMin=[]  IntegratorOutMax=[]  FilterOutMin=[]  FilterOutMax=[]  SumI1OutMin=[]  SumI1OutMax=[]  SumI2OutMin=[]  SumI2OutMax=[]  SumI3OutMin=[]  SumI3OutMax=[]  SumI4OutMin=[]  SumI4OutMax=[]  SumDOutMin=[]  SumDOutMax=[]  DifferentiatorOutMin=[]  DifferentiatorOutMax=[]  FilterDiffOutCoefMin=[]  FilterDiffOutCoefMax=[]  ReciprocalOutMin=[]  ReciprocalOutMax=[]  SumDenOutMin=[]  SumDenOutMax=[]  SumNumOutMin=[]  SumNumOutMax=[]  DivideOutMin=[]  DivideOutMax=[]  UdiffTsProdOutMin=[]  UdiffTsProdOutMax=[]  NTsProdOutMin=[]  NTsProdOutMax=[]  UintegralTsProdOutMin=[]  UintegralTsProdOutMax=[]  UngainTsProdOutMin=[]  UngainTsProdOutMax=[]  IntegratorContinuousStateAttributes=''  IntegratorStateMustResolveToSignalObject=off  IntegratorRTWStateStorageClass=Auto  FilterContinuousStateAttributes=''  FilterStateMustResolveToSignalObject=off  FilterRTWStateStorageClass=Auto  ParallelPVariant=Passthrough  IdealPVariant=InternalParameters  IVariant=InternalParameters  DVariant=Disabled  IntegratorVariant=Discrete  SatVariant=Enabled  AWVariant=Passthrough  PCopyVariant=Disabled  TRVariant=Disabled  FdbkBlocksVariant=Forward  IdealPFdbkVariant=Disabled  SatFdbkVariant=Disabled  DerivativeFilterVariant=Disabled  NVariant=Disabled  NCopyVariant=Disabled_SignalSpec  FilterICVariant=Disabled  IntegratorICVariant=InternalICs  ExternalResetVariant=Disabled  TRSumVariant=Passthrough  SumFdbkVariant=Disabled  SumVariant=Sum_PI  TsampFilterVariant=InternalTs  TsampNgainVariant=Passthrough  TsampIntegralVariant=Passthrough  ExternalSaturationOutDataTypeStr=Inherit: Same as second input
  Current Controller2 : pid_lib/PID Controller  Controller=PI  Form=Ideal  TimeDomain=Discrete-time  UseExternalTs=off  SampleTime=-1  IntegratorMethod=Forward Euler  FilterMethod=Forward Euler  ControllerParametersSource=internal  P=10  I=5  D=0  UseFilter=on  N=100  TunerSelectOption=Transfer Function Based (PID Tuner App)  InitialConditionSource=internal  InitialConditionForIntegrator=0  InitialConditionForFilter=0  DifferentiatorICPrevScaledInput=0  ExternalReset=none  TrackingMode=off  Kt=1  LimitOutput=on  SatLimitsSource=internal  UpperSaturationLimit=500  LowerSaturationLimit=-500  LinearizeAsGain=on  AntiWindupMode=none  Kb=1  POutMin=[]  POutMax=[]  IOutMin=[]  IOutMax=[]  DOutMin=[]  DOutMax=[]  NOutMin=[]  NOutMax=[]  SumOutMin=[]  SumOutMax=[]  SaturationOutMin=[]  SaturationOutMax=[]  PParamMin=[]  PParamMax=[]  IParamMin=[]  IParamMax=[]  DParamMin=[]  DParamMax=[]  NParamMin=[]  NParamMax=[]  KbParamMin=[]  KbParamMax=[]  KtParamMin=[]  KtParamMax=[]  KbOutMin=[]  KbOutMax=[]  KtOutMin=[]  KtOutMax=[]  IntegratorOutMin=[]  IntegratorOutMax=[]  FilterOutMin=[]  FilterOutMax=[]  SumI1OutMin=[]  SumI1OutMax=[]  SumI2OutMin=[]  SumI2OutMax=[]  SumI3OutMin=[]  SumI3OutMax=[]  SumI4OutMin=[]  SumI4OutMax=[]  SumDOutMin=[]  SumDOutMax=[]  DifferentiatorOutMin=[]  DifferentiatorOutMax=[]  FilterDiffOutCoefMin=[]  FilterDiffOutCoefMax=[]  ReciprocalOutMin=[]  ReciprocalOutMax=[]  SumDenOutMin=[]  SumDenOutMax=[]  SumNumOutMin=[]  SumNumOutMax=[]  DivideOutMin=[]  DivideOutMax=[]  UdiffTsProdOutMin=[]  UdiffTsProdOutMax=[]  NTsProdOutMin=[]  NTsProdOutMax=[]  UintegralTsProdOutMin=[]  UintegralTsProdOutMax=[]  UngainTsProdOutMin=[]  UngainTsProdOutMax=[]  IntegratorContinuousStateAttributes=''  IntegratorStateMustResolveToSignalObject=off  IntegratorRTWStateStorageClass=Auto  FilterContinuousStateAttributes=''  FilterStateMustResolveToSignalObject=off  FilterRTWStateStorageClass=Auto  ParallelPVariant=Passthrough  IdealPVariant=InternalParameters  IVariant=InternalParameters  DVariant=Disabled  IntegratorVariant=Discrete  SatVariant=Enabled  AWVariant=Passthrough  PCopyVariant=Disabled  TRVariant=Disabled  FdbkBlocksVariant=Forward  IdealPFdbkVariant=Disabled  SatFdbkVariant=Disabled  DerivativeFilterVariant=Disabled  NVariant=Disabled  NCopyVariant=Disabled_SignalSpec  FilterICVariant=Disabled  IntegratorICVariant=InternalICs  ExternalResetVariant=Disabled  TRSumVariant=Passthrough  SumFdbkVariant=Disabled  SumVariant=Sum_PI  TsampFilterVariant=InternalTs  TsampNgainVariant=Passthrough  TsampIntegralVariant=Passthrough  ExternalSaturationOutDataTypeStr=Inherit: Same as second input
  Decoupler : Subsystem
  Scope4 : Scope  NumInputPorts=2
  Scope5 : Scope  NumInputPorts=2
  Scope7 : Scope  NumInputPorts=2
  Sum3 : Sum  Inputs=|+-
  Sum6 : Sum  Inputs=|+-
  wires:
  Current Controller1/1 -> Scope5/1, Decoupler/1(Vs_q')
  Current Controller2/1 -> Scope5/2, Decoupler/2(Vs_d')
  [i_sd] -> Sum6/2, Scope4/2
  Sum3/1 -> Current Controller1/1
  [i_sq] -> Scope7/2, Sum3/2
  Sum6/1 -> Current Controller2/1

== system NN Controlled IM Drive/Space Vector PWM based VSI /Gating Pulse Generator/Gate Pulse Generator for 0121 Sequence ==
  "S1, S3, S5, sector" : Inport
  AND{,1..5} (6 alike) : Logic  IconShape=distinctive  AllPortsSameDT=off  OutDataTypeStr=boolean
  Constant : Constant  Value=2
  Data Type Conversion : DataTypeConversion
  Demux : Demux
  For Even Sector : Subsystem
  For Odd Sector : Subsystem
  Mod : Math  Operator=mod  SaturateOnIntegerOverflow=on
  Mux : Mux  Inputs=3
  NOT : Logic  Operator=NOT  IconShape=distinctive  AllPortsSameDT=off  OutDataTypeStr=boolean
  OR : Logic  Operator=OR  IconShape=distinctive  AllPortsSameDT=off  OutDataTypeStr=boolean
  OR1 : Logic  Operator=OR  IconShape=distinctive  AllPortsSameDT=off  OutDataTypeStr=boolean
  OR2 : Logic  Operator=OR  IconShape=distinctive  AllPortsSameDT=off  OutDataTypeStr=boolean
  Scope1 : Scope  NumInputPorts=4
  Gate 1 Pulse : Outport
  Gate 3 Pulse : Outport  Port=2
  Gate 5 Pulse : Outport  Port=3
  wires:
  For Odd Sector/3(Gate 5 Pulse) -> AND5/1
  OR2/1 -> Scope1/3, Gate 5 Pulse/1
  OR1/1 -> Scope1/2, Gate 3 Pulse/1
  Demux/3 -> Mux/3
  AND4/1 -> OR1/1
  OR/1 -> Scope1/1, Gate 1 Pulse/1
  For Odd Sector/1(Gate 1 Pulse) -> AND3/1
  AND5/1 -> OR2/1
  Demux/2 -> Mux/2
  AND1/1 -> OR1/2
  AND/1 -> OR/2
  Demux/4 -> Scope1/4, Mod/1
  For Even Sector/3(Gate 5 Pulse) -> AND2/1
  For Odd Sector/2(Gate 3 Pulse) -> AND4/1
  For Even Sector/1(Gate 1 Pulse) -> AND/1
  Data Type Conversion/1 -> AND3/2, AND4/2, AND5/2, NOT/1
  AND2/1 -> OR2/2
  Demux/1 -> Mux/1
  Mux/1 -> For Even Sector/1("S1, S3, S5"), For Odd Sector/1("S1, S3, S5")
  For Even Sector/2(Gate 3 Pulse) -> AND1/1
  Constant/1 -> Mod/2
  NOT/1 -> AND/2, AND1/2, AND2/2
  Mod/1 -> Data Type Conversion/1
  "S1, S3, S5, sector"/1 -> Demux/1
  AND3/1 -> OR/1

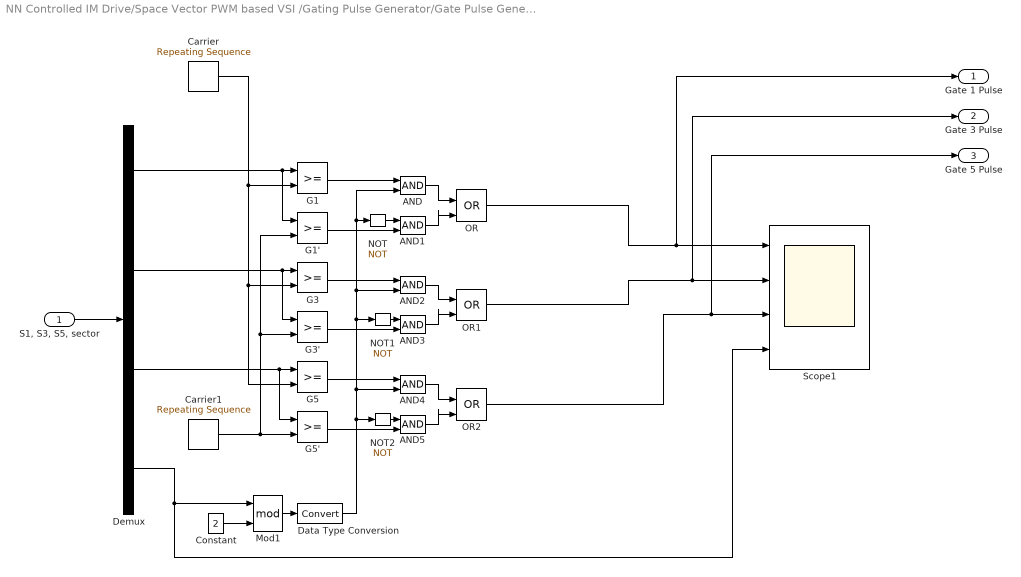
== system NN Controlled IM Drive/Space Vector PWM based VSI /Gating Pulse Generator/Gate Pulse Generator for 0127 Sequence ==
  "S1, S3, S5, sector" : Inport
  AND{,1..5} (6 alike) : Logic  IconShape=distinctive  AllPortsSameDT=off  OutDataTypeStr=boolean
  Carrier : simulink/Sources/Repeating Sequence  rep_seq_t=[0 Ts/2 Ts]  rep_seq_y=[Ts-(1e-16) 0 Ts-(1e-16)]
  Carrier1 : simulink/Sources/Repeating Sequence  rep_seq_t=[0 Ts/2 Ts]  rep_seq_y=[0 Ts-(1e-16) 0]
  Constant : Constant  Value=2
  Data Type Conversion : DataTypeConversion
  Demux : Demux
  G1 : RelationalOperator  OutDataTypeStr=boolean  RndMeth=Simplest
  G1' : RelationalOperator  OutDataTypeStr=boolean  RndMeth=Simplest
  G3 : RelationalOperator  OutDataTypeStr=boolean  RndMeth=Simplest
  G3' : RelationalOperator  OutDataTypeStr=boolean  RndMeth=Simplest
  G5 : RelationalOperator  OutDataTypeStr=boolean  RndMeth=Simplest
  G5' : RelationalOperator  OutDataTypeStr=boolean  RndMeth=Simplest
  Mod1 : Math  Operator=mod  SaturateOnIntegerOverflow=on
  NOT : Logic  Operator=NOT  IconShape=distinctive  AllPortsSameDT=off  OutDataTypeStr=boolean
  NOT1 : Logic  Operator=NOT  IconShape=distinctive  AllPortsSameDT=off  OutDataTypeStr=boolean
  NOT2 : Logic  Operator=NOT  IconShape=distinctive  AllPortsSameDT=off  OutDataTypeStr=boolean
  OR : Logic  Operator=OR  IconShape=distinctive  AllPortsSameDT=off  OutDataTypeStr=boolean
  OR1 : Logic  Operator=OR  IconShape=distinctive  AllPortsSameDT=off  OutDataTypeStr=boolean
  OR2 : Logic  Operator=OR  IconShape=distinctive  AllPortsSameDT=off  OutDataTypeStr=boolean
  Scope1 : Scope  NumInputPorts=4
  Gate 1 Pulse : Outport
  Gate 3 Pulse : Outport  Port=2
  Gate 5 Pulse : Outport  Port=3
  wires:
  G3/1 -> AND2/1
  OR2/1 -> Gate 5 Pulse/1, Scope1/3
  G3'/1 -> AND3/2
  OR/1 -> Gate 1 Pulse/1, Scope1/1
  Constant/1 -> Mod1/2
  AND1/1 -> OR/2
  Data Type Conversion/1 -> NOT2/1, AND4/2, NOT1/1, AND2/2, NOT/1, AND/2
  G5'/1 -> AND5/2
  G5/1 -> AND4/1
  AND5/1 -> OR2/2
  AND4/1 -> OR2/1
  AND/1 -> OR/1
  OR1/1 -> Scope1/2, Gate 3 Pulse/1
  NOT/1 -> AND1/1
  Mod1/1 -> Data Type Conversion/1
  AND3/1 -> OR1/2
  NOT2/1 -> AND5/1
  NOT1/1 -> AND3/1
  Carrier1/1 -> G1'/2, G3'/2, G5'/2
  Demux/1 -> G1'/1, G1/1
  G1'/1 -> AND1/2
  G1/1 -> AND/1
  Carrier/1 -> G5/2, G3/2, G1/2
  AND2/1 -> OR1/1
  "S1, S3, S5, sector"/1 -> Demux/1
  Demux/4 -> Scope1/4, Mod1/1
  Demux/2 -> G3'/1, G3/1
  Demux/3 -> G5'/1, G5/1

== system NN Controlled IM Drive/Space Vector PWM based VSI /Gating Pulse Generator/Gate Pulse Generator for 0127 Sequence 1 ==
  "S1, S3, S5, sector" : Inport
  AND{,1..5} (6 alike) : Logic  IconShape=distinctive  AllPortsSameDT=off  OutDataTypeStr=boolean
  Constant : Constant  Value=2
  Data Type Conversion : DataTypeConversion
  Demux : Demux
  For Even Sector : Subsystem
  For Odd Sector : Subsystem
  Mod : Math  Operator=mod  SaturateOnIntegerOverflow=on
  Mux : Mux  Inputs=3
  NOT : Logic  Operator=NOT  IconShape=distinctive  AllPortsSameDT=off  OutDataTypeStr=boolean
  OR : Logic  Operator=OR  IconShape=distinctive  AllPortsSameDT=off  OutDataTypeStr=boolean
  OR1 : Logic  Operator=OR  IconShape=distinctive  AllPortsSameDT=off  OutDataTypeStr=boolean
  OR2 : Logic  Operator=OR  IconShape=distinctive  AllPortsSameDT=off  OutDataTypeStr=boolean
  Scope1 : Scope  NumInputPorts=4
  Gate 1 Pulse : Outport
  Gate 3 Pulse : Outport  Port=2
  Gate 5 Pulse : Outport  Port=3
  wires:
  "S1, S3, S5, sector"/1 -> Demux/1
  Demux/1 -> Mux/1
  Demux/2 -> Mux/2
  Demux/3 -> Mux/3
  Mux/1 -> For Even Sector/1("S1, S3, S5"), For Odd Sector/1("S1, S3, S1")
  Demux/4 -> Scope1/4, Mod/1
  Constant/1 -> Mod/2
  Mod/1 -> Data Type Conversion/1
  NOT/1 -> AND/2, AND1/2, AND2/2
  For Odd Sector/1(Gate 1 Pulse1) -> AND3/1
  Data Type Conversion/1 -> AND3/2, AND4/2, AND5/2, NOT/1
  AND3/1 -> OR/1
  AND/1 -> OR/2
  AND4/1 -> OR1/1
  AND1/1 -> OR1/2
  AND5/1 -> OR2/1
  AND2/1 -> OR2/2
  OR1/1 -> Scope1/2, Gate 3 Pulse/1
  OR/1 -> Scope1/1, Gate 1 Pulse/1
  OR2/1 -> Scope1/3, Gate 5 Pulse/1
  For Even Sector/1(Gate 1 Pulse) -> AND/1
  For Even Sector/2(Gate 3 Pulse) -> AND1/1
  For Even Sector/3(Gate 5 Pulse) -> AND2/1
  For Odd Sector/2(Gate 3 Pulse1) -> AND4/1
  For Odd Sector/3(Gate 5 Pulse1) -> AND5/1
